simulink model "digital_scale"  (R2024b)
settings: Solver=VariableStepAuto  StartTime=0.0  StopTime=10.0  RelTol=1e-3
values from neighbouring files (symbols this model uses):
  c = 1500    [parameters.m]
  d = 8.5    [parameters.m]
  g = 9.81    [parameters.m]
  KG = 5    [parameters.m]
  L = 20    [parameters.m]
  m = 0.02    [parameters.m]
  mp = 0.03    [parameters.m]
  R = 1    [parameters.m]
  v0 = 0    [parameters.m]
  x0 = 0    [parameters.m]
settings Model: Creator=kavin  LastModifiedBy=kavin

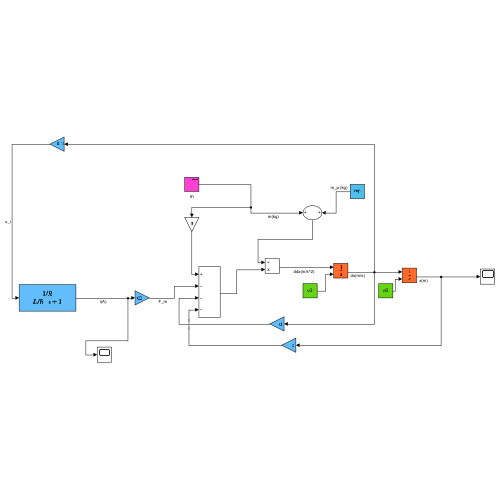
[thumbnail: Simulink's stored preview of the top-level diagram]
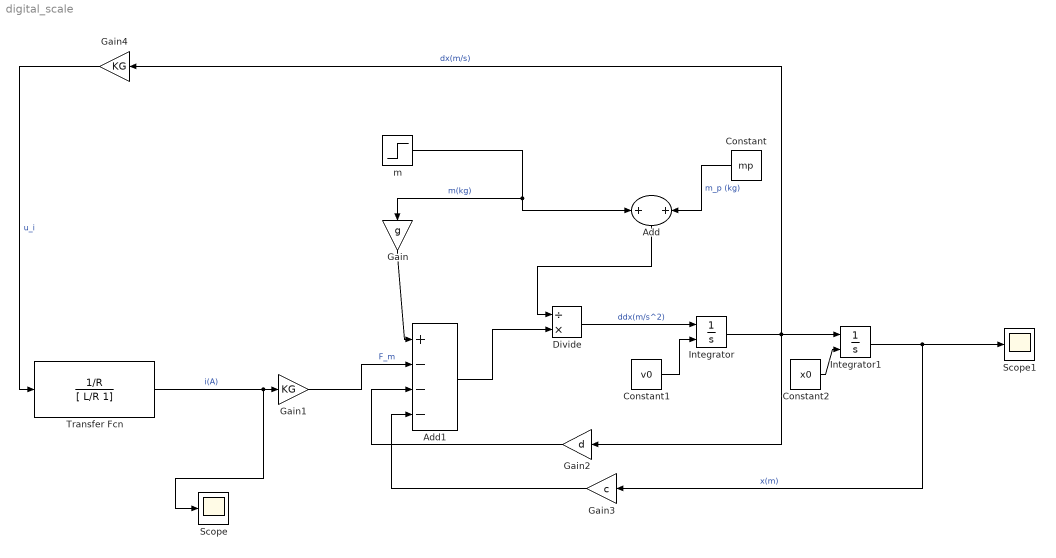
== system digital_scale ==
  Add : Sum
  Add1 : Sum  Inputs=+---
  Constant : Constant  Value=mp
  Constant1 : Constant  Value=v0
  Constant2 : Constant  Value=x0
  Divide : Product  Inputs=/*
  Gain : Gain  Gain=g
  Gain1 : Gain  Gain=KG
  Gain2 : Gain  Gain=d
  Gain3 : Gain  Gain=c
  Gain4 : Gain  Gain=KG
  Integrator : Integrator  InitialConditionSource=external
  Integrator1 : Integrator  InitialConditionSource=external
  Scope : Scope
  Scope1 : Scope
  Transfer Fcn : TransferFcn  Numerator=1/R  Denominator=[ L/R 1]
  m : Step  After=m  SampleTime=0
  wires:
  Constant2/1 -> Integrator1/2
  Constant1/1 -> Integrator/2
  Integrator/1 -> Gain4/1, Gain2/1, Integrator1/1  "dx(m/s)"
  Divide/1 -> Integrator/1  "ddx(m/s^2)"
  Integrator1/1 -> Gain3/1, Scope1/1  "x(m)"
  Transfer Fcn/1 -> Scope/1, Gain1/1  "i(A)"
  Constant/1 -> Add/2  "m_p (kg)"
  m/1 -> Gain/1, Add/1  "m(kg)"
  Add/1 -> Divide/1
  Add1/1 -> Divide/2
  Gain/1 -> Add1/1
  Gain1/1 -> Add1/2  "F_m"
  Gain2/1 -> Add1/3
  Gain3/1 -> Add1/4
  Gain4/1 -> Transfer Fcn/1  "u_i"
